simulink model "gtobuck_idealswitching"  (R2014a)
settings: Solver=ode23tb  SolverMode=SingleTasking  StartTime=0.0  StopTime=0.2  RelTol=1e-4
PreLoadFcn:
  | warning('off','SimPowerSystems:powersolve:RecommendedSolver');
StartFcn:
  | tic;
StopFcn:
  | toc;
libraries: powerlib x14
Description:
  | Copyright 2008 The MathWorks(TM), Inc.
settings Model: ExtModeTrigMode=oneshot  ExtModeArmWhenConnect=off  ExtModeAutoUpdateStatusClock=off  Creator=patrice  LastModifiedBy=cosorio
settings DataIOCC: LimitDataPoints=off  DSMLogging=off  SaveTime=off  SignalLoggingName=sigsOut
settings OptimizationCC: BooleanDataType=off  ExpressionDepthLimit=2147483647  InitFltsAndDblsToZero=on  EfficientMapNaN2IntZero=off
settings DebuggingCC: SaveWithParameterizedLinksMsg=none  UnderspecifiedInitializationDetection=Classic  SignalResolutionControl=TryResolveAllWithWarning  SolverPrmCheckMsg=none  MultiTaskDSMMsg=warning  MultiTaskCondExecSysMsg=none  FcnCallInpInsideContextMsg=UseLocalSettings  StateNameClashWarn=warning
settings HardwareCC: TargetUnknown=on
settings RTWCC: IncludeERTFirstTime=on
settings GRTTargetCC: TargetFcnLib=ansi_tfl_tmw.mat  CombineOutputUpdateFcns=off  GRTInterface=on

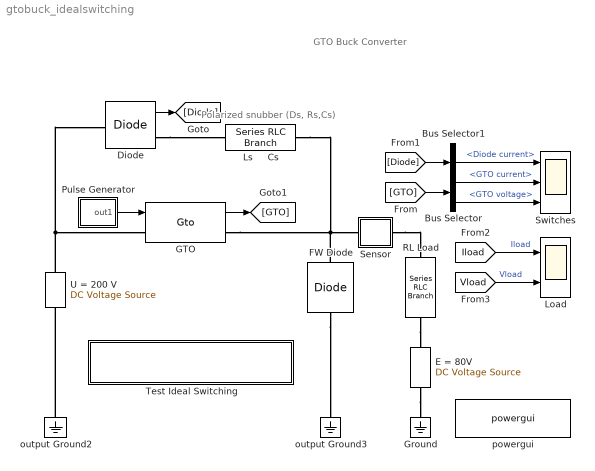
== system gtobuck_idealswitching ==
  note: GTO Buck Converter
  note: Polarized snubber (Ds, Rs,Cs)
  Bus Selector : BusSelector  OutputSignals=GTO current,GTO voltage
  Bus Selector1 : BusSelector  OutputSignals=Diode current
  Diode : powerlib/Power Electronics/Diode  Ron=0.01  Lon=0  Vf=0.8  IC=0  UseSnubber=off  Rs=100  Cs=Inf  Measurements=on
  E = 80V : powerlib/Electrical Sources/DC Voltage Source  Description=source block  Amplitude=80  Measurements=None
      settings: AttributesFormatString=\n
  FW Diode : powerlib/Power Electronics/Diode  Ron=0.01  Lon=0  Vf=0.8  IC=0  UseSnubber=off  Rs=100  Cs=0.1e-6  Measurements=off
  GTO : powerlib/Power Electronics/Gto  Ron=0.01  Lon=0  Vf=1  Tf=5e-6  Tt=10e-6  IC=0  Rs=inf  Cs=0  Measurements=on
      settings: AttributesFormatString=\n
  Ground : powerlib/Elements/Ground  LConnTagsString=a
  Load : Scope  NumInputPorts=2
      settings: YMin=-20~-50  YMax=60~250  MaxDataPoints=500000
  Ls     Cs : powerlib/Elements/Series RLC Branch  LConnTagsString=__new0  RConnTagsString=__new0  BranchType=LC  Resistance=1.0  Inductance=5e-7  SetiL0=off  InitialCurrent=0  Capacitance=2e-6  Setx0=off  InitialVoltage=0  Measurements=None
  Pulse Generator : Subsystem  mask(Pulse Generator){period=1e-3, duty=60, amplitude=1, start=0.5e-3}
      mask prompts: period "Period (secs):"; duty "Duty cycle (% of period):"; start "Start time:"
      mask help: Pulse Generator
      mask Help: Pulse generator which ensures pulse transitions are hit. Provides a vector of pulses when the height is entered as a vector.  Unmask to see how it works.
      mask Display: plot(0,0,100,100,[95,90,90,75,75,60,60,45,45,30,30,15,15,5],[25,25,75,75,25,25,75,75,25,25,75,75,25,25]);
  RL Load : powerlib/Elements/Series RLC Branch  LConnTagsString=__new0  RConnTagsString=__new0  BranchType=RL  Resistance=1  Inductance=5e-03  SetiL0=off  InitialCurrent=0  Capacitance=1.0  Setx0=off  InitialVoltage=0  Measurements=None
  Sensor : Subsystem
  Switches : Scope  NumInputPorts=3
      settings: YMin=0~0~0  YMax=60~60~300  SaveName=GTO_Data  MaxDataPoints=500000
  Test Ideal Switching : Subsystem
      settings: OpenFcn=compare_idealswitching
      mask Display: disp('Double click here to compare\nSwitching algorithms')
  U = 200 V : powerlib/Electrical Sources/DC Voltage Source  Description=source block  Amplitude=200  Measurements=None
      settings: AttributesFormatString=\n
  output Ground2 : powerlib/Elements/Ground  LConnTagsString=a
  output Ground3 : powerlib/Elements/Ground  LConnTagsString=a
  powergui : powerlib/powergui  Priority=2  SimulationMode=Continuous  SolverType=Tustin  SampleTime=1e-6  frequency=60  SPID=off  DisableSnubberDevices=on  DisableRonSwitches=off  DisableVfSwitches=off  SwTol=0  Interpol=off  DisplayEquations=off  Ts=0  methode=off  frequencyindice=0  Pbase=100e6  ErrMax=1e-4  Iterations=50  UnitsV=kV  UnitsW=MW  FunctionMessages=off  echomessages=off  HookPort=off  EnableUseOfTLC=off  x0status=blocks  RestoreLinks=warning  ResistiveCurrentMeasurement=off  Frange=[0:2:500]  Ylog=off  Xlog=on  ShowGrid=off  save=off  variable=ZData  structure=0  ZoomFFT=on  StartTime=0.0  cycles=1  DisplayStyle=1  fundamental=60  FreqAxis=off  MaxFrequency=1000  frequencyindicesteady=1  RmsSteady=1  display=off
  wires:
  Pulse Generator/1(out1) -> GTO/1
  Bus Selector/1 -> Switches/2  "<GTO current>"
  Bus Selector/2 -> Switches/3  "<GTO voltage>"
  Bus Selector1/1 -> Switches/1  "<Diode current>"
  Diode/1 -> [Diode]
  GTO/1 -> [GTO]
  [GTO] -> Bus Selector/1
  [Diode] -> Bus Selector1/1
  [Iload] -> Load/1  "Iload"
  [Vload] -> Load/2  "Vload"
  connections:
  Diode/RConn1 -- Ls     Cs/LConn1
  Sensor/RConn1 -- RL Load/LConn1
  FW Diode/LConn1 -- output Ground3/LConn1
  E = 80V/LConn1 -- Ground/LConn1
  RL Load/RConn1 -- E = 80V/RConn1
  U = 200 V/RConn1 -- GTO/LConn1 -- Diode/LConn1
  output Ground2/LConn1 -- U = 200 V/LConn1
  Ls     Cs/RConn1 -- Sensor/LConn1 -- FW Diode/RConn1 -- GTO/RConn1

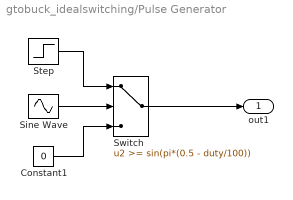
== system gtobuck_idealswitching/Pulse Generator ==
  Constant1 : Constant  Value=0
  Sine Wave : Sin  Frequency=2*pi./period  Phase=-2*pi*(start./period + duty/200 - 1/4)  SampleTime=0
  Step : Step  Time=start  After=amplitude  SampleTime=0
  Switch : Switch  Threshold=sin(pi*(0.5 - duty/100))  SaturateOnIntegerOverflow=on  InputSameDT=on
  out1 : Outport  InitialOutput=0
  wires:
  Step/1 -> Switch/1
  Constant1/1 -> Switch/3
  Switch/1 -> out1/1
  Sine Wave/1 -> Switch/2

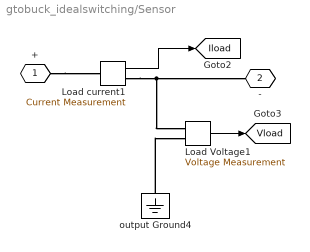
== system gtobuck_idealswitching/Sensor ==
  Load Voltage1 : powerlib/Measurements/Voltage Measurement  Tag=PoWeRsYsTeMmEaSuReMeNt  PhasorSimulation=off  OutputType=Magnitude  PSBequivalent=0
  Load current1 : powerlib/Measurements/Current Measurement  Tag=PoWeRsYsTeMmEaSuReMeNt  PhasorSimulation=off  OutputType=Magnitude  PSBequivalent=0
  output Ground4 : powerlib/Elements/Ground  LConnTagsString=a
  + : PMIOPort  Tag=PMCPort  Port=1  Side=Left
  - : PMIOPort  Tag=PMCPort  Port=2  Side=Right
  tag scope: Iload=global, Vload=global
  wires:
  Load current1/1 -> [Iload]
  Load Voltage1/1 -> [Vload]
  connections:
  output Ground4/LConn1 -- Load Voltage1/LConn2
  +/RConn1 -- Load current1/LConn1
  Load current1/RConn1 -- Load Voltage1/LConn1 -- -/RConn1

== system gtobuck_idealswitching/Test Ideal Switching ==
  note: 22X Speedup with Ideal Switching!
